simulink model "txPacketGenerator"  (R2022a)
settings: Solver=FixedStepDiscrete  StartTime=0.0  StopTime=simTime  RelTol=1e-3
libraries: dspsrcs4 x8
settings Model: DataTypeOverride=Off  Creator=alpha  LastModifiedBy=alpha
settings SolverCC: AlgebraicLoopSolver=TrustRegion
settings DataIOCC: LimitDataPoints=on  SaveOutput=off  SaveTime=off
settings OptimizationCC: BlockReduction=off  ConditionallyExecuteInputs=off  DefaultParameterBehavior=Inlined  LifeSpan=inf
settings DebuggingCC: AlgebraicLoopMsg=error  SingleTaskRateTransMsg=error  UnconnectedInputMsg=warning  UnconnectedOutputMsg=warning  UnconnectedLineMsg=warning  AllowSymbolicDim=off  StrictBusMsg=ErrorOnBusTreatedAsVector  SFUnexpectedBacktrackingDiag=warning  SFNoUnconditionalDefaultTransitionDiag=warning  SFExecutionAtInitializationDiag=none  SFMachineParentedDataDiag=warning  ArithmeticOperatorsInVariantConditions=warning
settings HardwareCC: ProdBitPerPointer=32  ProdBitPerSizeT=32  ProdBitPerPtrDiffT=32  ProdLargestAtomicFloat=None  ProdIntDivRoundTo=Undefined  ProdEndianess=Unspecified  ProdWordSize=32  ProdHWDeviceType=ASIC/FPGA->ASIC/FPGA  ProdEqTarget=off
settings SFSimCC: SimUseLocalCustomCode=off  CustomCodeUndefinedFunction=UseInterfaceOnly
settings RTWCC: RTWUseLocalCustomCode=off
settings CodeAppCC: StateflowObjectComments=on
settings GRTTargetCC: TargetLangStandard=C89/C90 (ANSI)
settings ConfigComp: CovScope=ReferencedModels  CovMetricSettings=dw  CovSaveCumulativeToWorkspaceVar=on  CovSaveSingleToWorkspaceVar=on  CovExternalEMLEnable=off  CovSFcnEnable=off

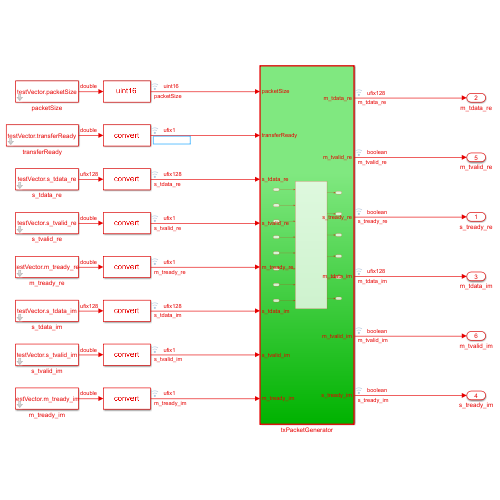
[thumbnail: Simulink's stored preview of the top-level diagram]
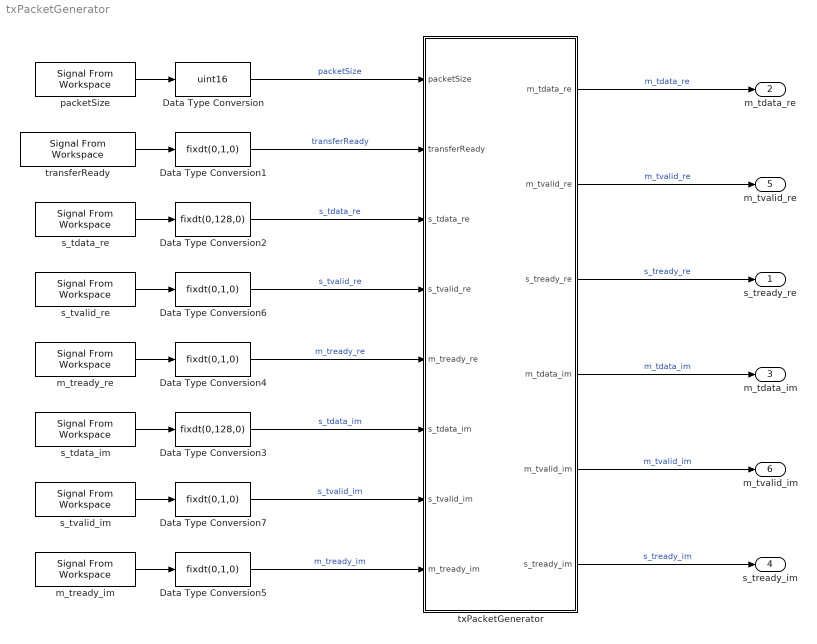
== system txPacketGenerator ==
  Data Type Conversion : DataTypeConversion  OutDataTypeStr=uint16  SaturateOnIntegerOverflow=off  RndMeth=Floor
  Data Type Conversion{1,4..7} (5 alike) : DataTypeConversion  OutDataTypeStr=fixdt(0,1,0)  SaturateOnIntegerOverflow=off  RndMeth=Floor
  Data Type Conversion2 : DataTypeConversion  OutDataTypeStr=fixdt(0,128,0)  SaturateOnIntegerOverflow=off  RndMeth=Floor
  Data Type Conversion3 : DataTypeConversion  OutDataTypeStr=fixdt(0,128,0)  SaturateOnIntegerOverflow=off  RndMeth=Floor
  m_tready_im : dspsrcs4/Signal From Workspace  X=testVector.m_tready_im  Ts=1  nsamps=1  OutputAfterFinalValue=Setting to zero  ignoreOrWarnInputAndFrameLengths=off  OutputFrames=off
  m_tready_re : dspsrcs4/Signal From Workspace  X=testVector.m_tready_re  Ts=1  nsamps=1  OutputAfterFinalValue=Setting to zero  ignoreOrWarnInputAndFrameLengths=off  OutputFrames=off
  packetSize : dspsrcs4/Signal From Workspace  X=testVector.packetSize  Ts=1  nsamps=1  OutputAfterFinalValue=Setting to zero  ignoreOrWarnInputAndFrameLengths=off  OutputFrames=off
  s_tdata_im : dspsrcs4/Signal From Workspace  X=testVector.s_tdata_im  Ts=1  nsamps=1  OutputAfterFinalValue=Setting to zero  ignoreOrWarnInputAndFrameLengths=off  OutputFrames=off
  s_tdata_re : dspsrcs4/Signal From Workspace  X=testVector.s_tdata_re  Ts=1  nsamps=1  OutputAfterFinalValue=Setting to zero  ignoreOrWarnInputAndFrameLengths=off  OutputFrames=off
  s_tvalid_im : dspsrcs4/Signal From Workspace  X=testVector.s_tvalid_im  Ts=1  nsamps=1  OutputAfterFinalValue=Setting to zero  ignoreOrWarnInputAndFrameLengths=off  OutputFrames=off
  s_tvalid_re : dspsrcs4/Signal From Workspace  X=testVector.s_tvalid_re  Ts=1  nsamps=1  OutputAfterFinalValue=Setting to zero  ignoreOrWarnInputAndFrameLengths=off  OutputFrames=off
  transferReady : dspsrcs4/Signal From Workspace  X=testVector.transferReady  Ts=1  nsamps=1  OutputAfterFinalValue=Setting to zero  ignoreOrWarnInputAndFrameLengths=off  OutputFrames=off
  txPacketGenerator : Subsystem  TreatAsAtomicUnit=on
  s_tready_re : Outport
  m_tdata_re : Outport  Port=2
  m_tdata_im : Outport  Port=3
  s_tready_im : Outport  Port=4
  m_tvalid_re : Outport  Port=5
  m_tvalid_im : Outport  Port=6
  wires:
  m_tready_im/1 -> Data Type Conversion5/1
  m_tready_re/1 -> Data Type Conversion4/1
  Data Type Conversion5/1 -> txPacketGenerator/8(m_tready_im)  "m_tready_im"
  Data Type Conversion4/1 -> txPacketGenerator/5(m_tready_re)  "m_tready_re"
  packetSize/1 -> Data Type Conversion/1
  txPacketGenerator/3(s_tready_re) -> s_tready_re/1  "s_tready_re"
  Data Type Conversion/1 -> txPacketGenerator/1(packetSize)  "packetSize"
  Data Type Conversion1/1 -> txPacketGenerator/2(transferReady)  "transferReady"
  txPacketGenerator/1(m_tdata_re) -> m_tdata_re/1  "m_tdata_re"
  Data Type Conversion3/1 -> txPacketGenerator/6(s_tdata_im)  "s_tdata_im"
  Data Type Conversion2/1 -> txPacketGenerator/3(s_tdata_re)  "s_tdata_re"
  s_tdata_re/1 -> Data Type Conversion2/1
  transferReady/1 -> Data Type Conversion1/1
  txPacketGenerator/4(m_tdata_im) -> m_tdata_im/1  "m_tdata_im"
  s_tvalid_re/1 -> Data Type Conversion6/1
  s_tvalid_im/1 -> Data Type Conversion7/1
  Data Type Conversion6/1 -> txPacketGenerator/4(s_tvalid_re)  "s_tvalid_re"
  Data Type Conversion7/1 -> txPacketGenerator/7(s_tvalid_im)  "s_tvalid_im"
  txPacketGenerator/2(m_tvalid_re) -> m_tvalid_re/1  "m_tvalid_re"
  txPacketGenerator/6(s_tready_im) -> s_tready_im/1  "s_tready_im"
  s_tdata_im/1 -> Data Type Conversion3/1
  txPacketGenerator/5(m_tvalid_im) -> m_tvalid_im/1  "m_tvalid_im"

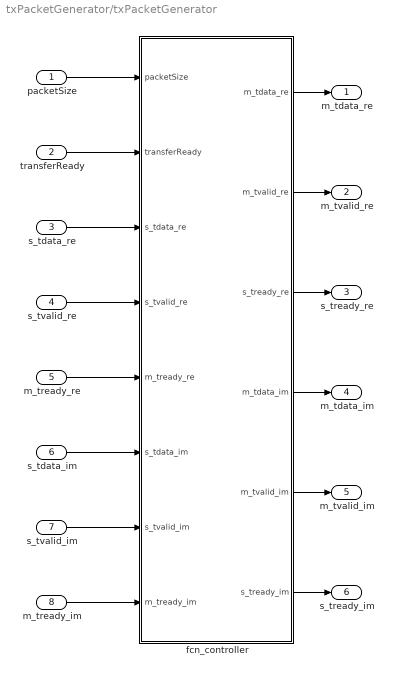
== system txPacketGenerator/txPacketGenerator ==
  packetSize : Inport
  transferReady : Inport  Port=2
  s_tdata_re : Inport  Port=3
  s_tvalid_re : Inport  Port=4
  m_tready_re : Inport  Port=5
  s_tdata_im : Inport  Port=6
  s_tvalid_im : Inport  Port=7
  m_tready_im : Inport  Port=8
  fcn_controller : MATLAB Function  TreatAsAtomicUnit=on
  m_tdata_re : Outport
  m_tvalid_re : Outport  Port=2
  s_tready_re : Outport  Port=3
  m_tdata_im : Outport  Port=4
  m_tvalid_im : Outport  Port=5
  s_tready_im : Outport  Port=6
  wires:
  m_tready_im/1 -> fcn_controller/8(m_tready_im)
  fcn_controller/5(m_tvalid_im) -> m_tvalid_im/1
  fcn_controller/2(m_tvalid_re) -> m_tvalid_re/1
  fcn_controller/1(m_tdata_re) -> m_tdata_re/1
  m_tready_re/1 -> fcn_controller/5(m_tready_re)
  s_tvalid_re/1 -> fcn_controller/4(s_tvalid_re)
  packetSize/1 -> fcn_controller/1(packetSize)
  fcn_controller/6(s_tready_im) -> s_tready_im/1
  transferReady/1 -> fcn_controller/2(transferReady)
  fcn_controller/3(s_tready_re) -> s_tready_re/1
  s_tdata_im/1 -> fcn_controller/6(s_tdata_im)
  s_tdata_re/1 -> fcn_controller/3(s_tdata_re)
  fcn_controller/4(m_tdata_im) -> m_tdata_im/1
  s_tvalid_im/1 -> fcn_controller/7(s_tvalid_im)

== matlab function txPacketGenerator/fcn_controller ==
  data: m_tdata_re output; m_tvalid_re output; packetSize input; transferReady input; s_tdata_re input; s_tvalid_re input; m_tready_re input; s_tready_re output; m_tdata_im output; m_tvalid_im output; s_tready_im output; s_tdata_im input; s_tvalid_im input; m_tready_im input
function [m_tdata_re, m_tvalid_re, s_tready_re, m_tdata_im, m_tvalid_im, s_tready_im]  = fcn_controller(packetSize, transferReady, ...
                                                                                s_tdata_re,  s_tvalid_re, m_tready_re,...
                                                                                s_tdata_im, s_tvalid_im, m_tready_im)
    %% Initialize Registers
    persistent counter_reg_re;
    if isempty(counter_reg_re)
        counter_reg_re = uint16(0);
    end  

    persistent counter_reg_im;
    if isempty(counter_reg_im)
        counter_reg_im = uint16(0);
    end     

    persistent state_reg_re;
    if isempty(state_reg_re)
        state_reg_re = fi(0,0,1,0);
    end  

    persistent state_reg_im;
    if isempty(state_reg_im)
        state_reg_im = fi(0,0,1,0);
    end      

    persistent transferReady_reg;
    if isempty(transferReady_reg)
        transferReady_reg = fi(0,0,1,0);
    end      

    %% Set outputs
    m_tvalid_re = state_reg_re == fi(1,0,1,0) && s_tvalid_re == fi(1,0,1,0);
    s_tready_re = state_reg_re == fi(1,0,1,0) && m_tready_re == fi(1,0,1,0);
    if state_reg_re == fi(1,0,1,0) && s_tvalid_re == fi(1,0,1,0)
        m_tdata_re = s_tdata_re;
    else
        m_tdata_re = fi(0,0,128,0);
    end
    
    m_tvalid_im = state_reg_im == fi(1,0,1,0) && s_tvalid_im == fi(1,0,1,0);
    s_tready_im = state_reg_im == fi(1,0,1,0) && m_tready_im == fi(1,0,1,0); 
    if state_reg_im == fi(1,0,1,0) && s_tvalid_im == fi(1,0,1,0)
        m_tdata_im = s_tdata_im;
    else
        m_tdata_im = fi(0,0,128,0);
    end
    
    transferReady_risingEdge = transferReady_reg == fi(0,0,1,0) && transferReady == fi(1,0,1,0);

    %% Update Registers
    switch state_reg_re
        case fi(0,0,1,0)
            if transferReady_risingEdge == 1 && packetSize>0
                state_reg_re = fi(1,0,1,0);
            end
            counter_reg_re = packetSize;
        case fi(1,0,1,0)
            if s_tvalid_re == fi(1,0,1,0) && m_tready_re == fi(1,0,1,0)
                if counter_reg_re == 1
                    state_reg_re = fi(0,0,1,0); 
                end
                counter_reg_re = counter_reg_re - 1;            
            end
    end

    switch state_reg_im
        case fi(0,0,1,0)
            if transferReady_risingEdge == 1 && packetSize>0
                state_reg_im = fi(1,0,1,0);
            end
            counter_reg_im = packetSize;
        case fi(1,0,1,0)
            if s_tvalid_im == fi(1,0,1,0) && m_tready_im == fi(1,0,1,0)
                if counter_reg_im == 1
                    state_reg_im = fi(0,0,1,0); 
                end
                counter_reg_im = counter_reg_im - 1;            
            end
    end    

    transferReady_reg = transferReady;
